simulink model "matrix5"  (R2018b)
settings: Solver=VariableStepAuto  StartTime=0.0  StopTime=1  RelTol=1e-6
model workspace (MAT data in the model file):
  A1 = 0.212
  A2 = 0.0033
  B1 = 0.311
  B2 = 0.0075
  C1 = 0.1
  C2 = 0.0084
  Ce1 = 0.27
  Ce2 = 0.12
  Cm1 = 0.36
  Cm2 = 0.12
  D1 = 0.1
  D2 = 0.001
  E1 = 0.1
  E2 = 0.001
  F1 = 0.1
  F2 = 0.001
  L1 = 0.00032
  L2 = 0.000194
  R1 = 0.32
  R2 = 0.485
  Xc2 = 0
  Yc2 = 0.0148
  g = 9.81
  m2 = 1.13085
settings Model: Creator=Sainquake  LastModifiedBy=Sainquake

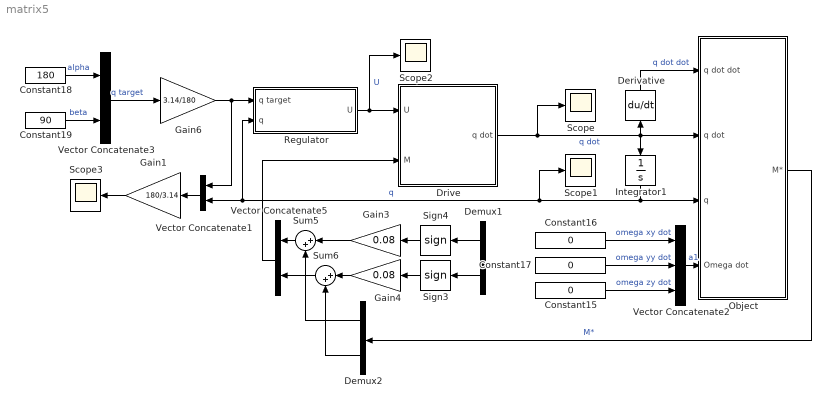
== system matrix5 ==
  Constant15 : Constant  Value=0
  Constant16 : Constant  Value=0
  Constant17 : Constant  Value=0
  Constant18 : Constant  Value=180
  Constant19 : Constant  Value=90
  Demux1 : Demux  Outputs=2
  Demux2 : Demux  Outputs=2
  Derivative : Derivative
  Drive : Subsystem
  Gain1 : Gain  Gain=180/3.14
  Gain3 : Gain  Gain=0.08
  Gain4 : Gain  Gain=0.08
  Gain6 : Gain  Gain=3.14/180
  Integrator1 : Integrator
  Object : Subsystem
  Regulator : Subsystem
  Scope{,1..3} (4 alike) : Scope
  Sign3 : Signum  ZeroCross=off
  Sign4 : Signum  ZeroCross=off
  Sum5 : Sum  Inputs=|++
  Sum6 : Sum  Inputs=|++
  Vector Concatenate1 : Concatenate
  Vector Concatenate2 : Concatenate  NumInputs=3
  Vector Concatenate3 : Concatenate
  Vector Concatenate5 : Concatenate
  wires:
  Integrator1/1 -> Regulator/2(q), Vector Concatenate1/2, Scope1/1, Object/3("q ")  "q"
  Constant15/1 -> Vector Concatenate2/3  "omega zy dot"
  Constant17/1 -> Vector Concatenate2/2  "omega yy dot"
  Constant16/1 -> Vector Concatenate2/1  "omega xy dot"
  Vector Concatenate2/1 -> Object/4(Omega dot)  "a1"
  Constant19/1 -> Vector Concatenate3/2  "beta"
  Constant18/1 -> Vector Concatenate3/1  "alpha"
  Drive/1(q dot) -> Integrator1/1, Object/2(q dot), Derivative/1, Scope/1  "q dot"
  Object/1(M*) -> Demux2/1  "M*"
  Regulator/1("U ") -> Scope2/1, Drive/1(U)  "U"
  Sign4/1 -> Gain3/1
  Sign3/1 -> Gain4/1
  Vector Concatenate5/1 -> Drive/2(M)
  Gain3/1 -> Sum5/1
  Demux2/1 -> Sum5/2
  Gain4/1 -> Sum6/1
  Demux2/2 -> Sum6/2
  Sum5/1 -> Vector Concatenate5/1
  Sum6/1 -> Vector Concatenate5/2
  Demux1/2 -> Sign3/1
  Demux1/1 -> Sign4/1
  Derivative/1 -> Object/1(q dot dot)  "q dot dot"
  Vector Concatenate3/1 -> Gain6/1  "q target"
  Vector Concatenate1/1 -> Gain1/1
  Gain1/1 -> Scope3/1
  Gain6/1 -> Vector Concatenate1/1, Regulator/1(q target)

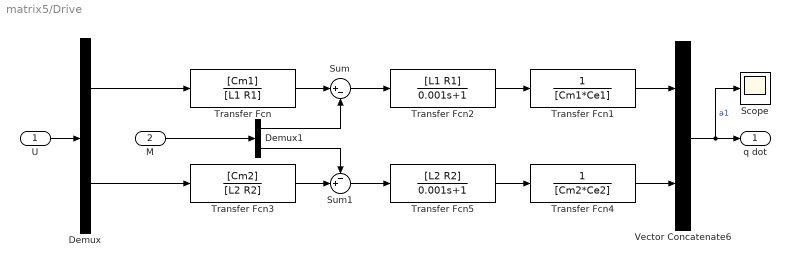
== system matrix5/Drive ==
  U : Inport
  M : Inport  Port=2
  Demux : Demux  Outputs=2
  Demux1 : Demux  Outputs=2
  Scope : Scope
  Sum : Sum  Inputs=|+-
  Sum1 : Sum  Inputs=-+|
  Transfer Fcn : TransferFcn  Numerator=[Cm1]  Denominator=[L1 R1]
  Transfer Fcn1 : TransferFcn  Numerator=1  Denominator=[Cm1*Ce1]
  Transfer Fcn2 : TransferFcn  Numerator=[L1 R1]  Denominator=[0.001 1]
  Transfer Fcn3 : TransferFcn  Numerator=[Cm2]  Denominator=[L2 R2]
  Transfer Fcn4 : TransferFcn  Numerator=1  Denominator=[Cm2*Ce2]
  Transfer Fcn5 : TransferFcn  Numerator=[L2 R2]  Denominator=[0.001 1]
  Vector Concatenate6 : Concatenate
  q dot : Outport
  wires:
  Sum/1 -> Transfer Fcn2/1
  Transfer Fcn3/1 -> Sum1/2
  Demux1/2 -> Sum1/1
  Demux/1 -> Transfer Fcn/1
  Vector Concatenate6/1 -> q dot/1, Scope/1  "a1"
  Transfer Fcn/1 -> Sum/1
  Transfer Fcn5/1 -> Transfer Fcn4/1
  Transfer Fcn2/1 -> Transfer Fcn1/1
  Demux1/1 -> Sum/2
  Demux/2 -> Transfer Fcn3/1
  Sum1/1 -> Transfer Fcn5/1
  Transfer Fcn1/1 -> Vector Concatenate6/1
  Transfer Fcn4/1 -> Vector Concatenate6/2
  U/1 -> Demux/1
  M/1 -> Demux1/1

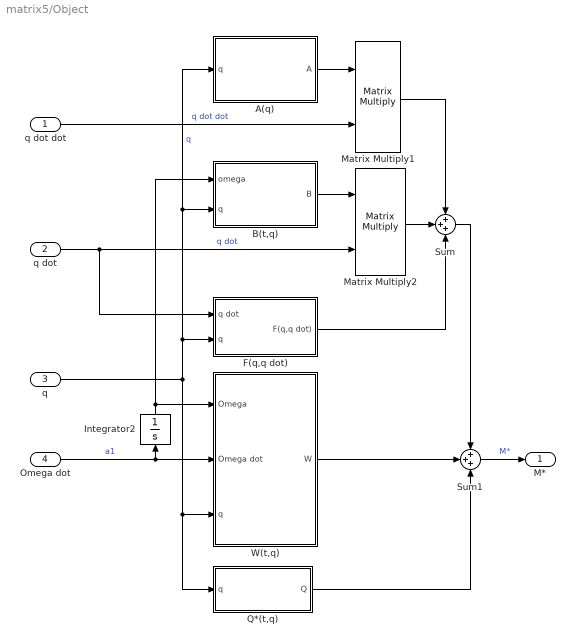
== system matrix5/Object ==
  q dot dot : Inport
  q dot : Inport  Port=2
  "q " : Inport  Port=3
  Omega dot : Inport  Port=4
  A(q) : Subsystem
  B(t,q) : Subsystem
  F(q,q dot) : Subsystem
  Integrator2 : Integrator
  Matrix Multiply1 : Product  Multiplication=Matrix(*)
  Matrix Multiply2 : Product  Multiplication=Matrix(*)
  Q*(t,q) : Subsystem
  Sum : Sum  Inputs=+++
  Sum1 : Sum  Inputs=+++
  W(t,q) : Subsystem
  M* : Outport
  wires:
  Integrator2/1 -> B(t,q)/1(omega), W(t,q)/1(Omega)
  Sum1/1 -> M*/1  "M*"
  A(q)/1(A) -> Matrix Multiply1/1
  q dot dot/1 -> Matrix Multiply1/2  "q dot dot"
  Omega dot/1 -> Integrator2/1, W(t,q)/2(Omega dot)  "a1"
  Sum/1 -> Sum1/1
  Matrix Multiply1/1 -> Sum/1
  Matrix Multiply2/1 -> Sum/2
  B(t,q)/1(B) -> Matrix Multiply2/1
  q dot/1 -> F(q,q dot)/1(q dot), Matrix Multiply2/2  "q dot"
  "q "/1 -> F(q,q dot)/2(q), B(t,q)/2(q), A(q)/1(q), Q*(t,q)/1(q), W(t,q)/3(q)  "q"
  W(t,q)/1(W) -> Sum1/2
  Q*(t,q)/1(Q) -> Sum1/3
  F(q,q dot)/1(F(q,q dot)) -> Sum/3

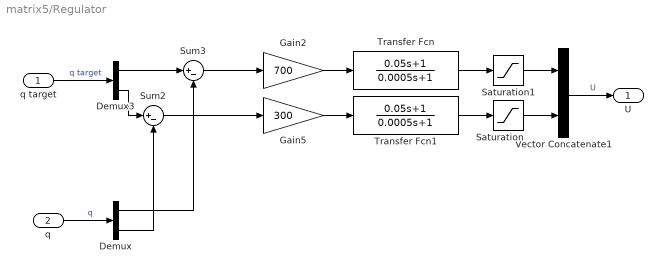
== system matrix5/Regulator ==
  q target : Inport
  q : Inport  Port=2
  Demux : Demux  Outputs=2
  Demux3 : Demux  Outputs=2
  Gain2 : Gain  Gain=700
  Gain5 : Gain  Gain=300
  Saturation : Saturate  UpperLimit=27  LowerLimit=-27  ZeroCross=off
  Saturation1 : Saturate  UpperLimit=27  LowerLimit=-27  ZeroCross=off
  Sum2 : Sum  Inputs=|+-
  Sum3 : Sum  Inputs=|+-
  Transfer Fcn : TransferFcn  Numerator=[0.05 1]  Denominator=[0.0005 1]
  Transfer Fcn1 : TransferFcn  Numerator=[0.05 1]  Denominator=[0.0005 1]
  Vector Concatenate1 : Concatenate
  "U " : Outport
  wires:
  Demux/1 -> Sum3/2
  Demux/2 -> Sum2/2
  Sum3/1 -> Gain2/1
  Transfer Fcn1/1 -> Saturation/1
  Saturation/1 -> Vector Concatenate1/2
  Sum2/1 -> Gain5/1
  Saturation1/1 -> Vector Concatenate1/1
  Demux3/2 -> Sum2/1
  Gain2/1 -> Transfer Fcn/1
  q target/1 -> Demux3/1  "q target"
  Gain5/1 -> Transfer Fcn1/1
  Demux3/1 -> Sum3/1
  Transfer Fcn/1 -> Saturation1/1
  q/1 -> Demux/1  "q"
  Vector Concatenate1/1 -> "U "/1  "U"

== system matrix5/Object/A(q) ==
  q : Inport
  B(beta) : Subsystem
  Constant10 : Constant  Value=C2
  Constant7 : Constant  Value=B1
  D(beta) : Subsystem
  Demux : Demux  Outputs=2
  Display5 : Display
  Gain : Gain  Gain=-1
  Sum : Sum  Inputs=|++
  Vector Concatenate1 : Concatenate
  Vector Concatenate2 : Concatenate
  Vector Concatenate6 : Concatenate  Mode=Multidimensional array  ConcatenateDimension=2
  A : Outport
  wires:
  q/1 -> Demux/1
  Constant7/1 -> Sum/2
  Vector Concatenate2/1 -> Vector Concatenate6/2  "a2"
  Sum/1 -> Vector Concatenate1/1  "a11"
  Constant10/1 -> Vector Concatenate2/2  "a22"
  Vector Concatenate1/1 -> Vector Concatenate6/1  "a1"
  B(beta)/1(B) -> Sum/1
  D(beta)/1(D) -> Gain/1
  Vector Concatenate6/1 -> A/1, Display5/1  "A"
  Gain/1 -> Vector Concatenate1/2, Vector Concatenate2/1  "a12"
  Demux/2 -> B(beta)/1(beta), D(beta)/1(beta)

== system matrix5/Object/B(t,q) ==
  omega : Inport
  q : Inport  Port=2
  Constant : Constant  Value=0
  Gain : Gain  Gain=-1
  Vector Concatenate3 : Concatenate
  Vector Concatenate4 : Concatenate
  Vector Concatenate5 : Concatenate  Mode=Multidimensional array  ConcatenateDimension=2
  b(t,alpha,beta) : Subsystem
  B : Outport
  wires:
  Vector Concatenate3/1 -> Vector Concatenate5/1  "a1"
  Vector Concatenate5/1 -> B/1  "A"
  Vector Concatenate4/1 -> Vector Concatenate5/2  "a2"
  b(t,alpha,beta)/1(b) -> Vector Concatenate3/2, Gain/1
  Gain/1 -> Vector Concatenate4/1
  Constant/1 -> Vector Concatenate4/2, Vector Concatenate3/1
  omega/1 -> b(t,alpha,beta)/1(omega)
  q/1 -> b(t,alpha,beta)/2(q)

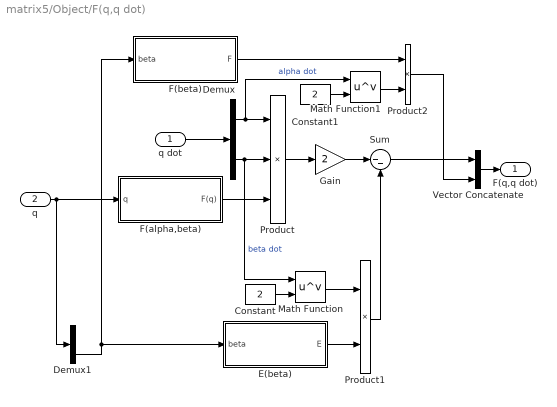
== system matrix5/Object/F(q,q dot) ==
  q dot : Inport
  q : Inport  Port=2
  Constant : Constant  Value=2
  Constant1 : Constant  Value=2
  Demux : Demux  Outputs=2
  Demux1 : Demux  Outputs=2
  E(beta) : Subsystem
  F(alpha,beta) : Subsystem
  F(beta) : Subsystem
  Gain : Gain  Gain=2
  Math Function : Math  Operator=pow  SaturateOnIntegerOverflow=on
  Math Function1 : Math  Operator=pow  SaturateOnIntegerOverflow=on
  Product : Product  Inputs=3
  Product1 : Product
  Product2 : Product
  Sum : Sum  Inputs=|--
  Vector Concatenate : Concatenate
  F(q,q dot) : Outport
  wires:
  q dot/1 -> Demux/1
  Product/1 -> Gain/1
  Demux/2 -> Product/2, Math Function/1  "beta dot"
  F(alpha,beta)/1(F(q)) -> Product/3
  q/1 -> Demux1/1, F(alpha,beta)/1(q)
  Constant/1 -> Math Function/2
  Math Function/1 -> Product1/1
  E(beta)/1(E) -> Product1/2
  Demux1/2 -> E(beta)/1(beta), F(beta)/1(beta)
  Gain/1 -> Sum/1
  Product1/1 -> Sum/2
  Constant1/1 -> Math Function1/2
  Demux/1 -> Product/1, Math Function1/1  "alpha dot"
  Math Function1/1 -> Product2/2
  F(beta)/1(F) -> Product2/1
  Product2/1 -> Vector Concatenate/2
  Sum/1 -> Vector Concatenate/1
  Vector Concatenate/1 -> F(q,q dot)/1

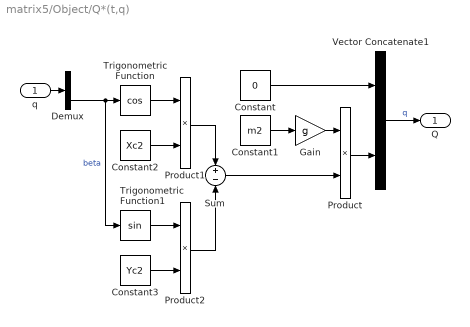
== system matrix5/Object/Q*(t,q) ==
  q : Inport
  Constant : Constant  Value=0
  Constant1 : Constant  Value=m2
  Constant2 : Constant  Value=Xc2
  Constant3 : Constant  Value=Yc2
  Demux : Demux  Outputs=2
  Gain : Gain  Gain=g
  Product : Product
  Product1 : Product
  Product2 : Product
  Sum : Sum  Inputs=+-
  Trigonometric Function : Trigonometry  Operator=cos
  Trigonometric Function1 : Trigonometry
  Vector Concatenate1 : Concatenate
  Q : Outport
  wires:
  Vector Concatenate1/1 -> Q/1  "q"
  Constant/1 -> Vector Concatenate1/1
  Product/1 -> Vector Concatenate1/2
  Gain/1 -> Product/1
  Constant1/1 -> Gain/1
  q/1 -> Demux/1
  Trigonometric Function/1 -> Product1/1
  Constant2/1 -> Product1/2
  Product1/1 -> Sum/1
  Constant3/1 -> Product2/2
  Demux/2 -> Trigonometric Function1/1, Trigonometric Function/1  "beta"
  Product2/1 -> Sum/2
  Trigonometric Function1/1 -> Product2/1
  Sum/1 -> Product/2

== system matrix5/Object/W(t,q) ==
  Omega : Inport
  Omega dot : Inport  Port=2
  q : Inport  Port=3
  Vector Concatenate : Concatenate
  "w alpha (t, q) " : Subsystem
  "w beta (t, q)" : Subsystem
  W : Outport
  wires:
  Omega/1 -> "w beta (t, q)"/1(Omega), "w alpha (t, q) "/1(Omega)
  Omega dot/1 -> "w beta (t, q)"/2(Omega dot), "w alpha (t, q) "/2(Omega dot)
  q/1 -> "w beta (t, q)"/3(q), "w alpha (t, q) "/3(q)
  "w alpha (t, q) "/1(w alpha) -> Vector Concatenate/1
  "w beta (t, q)"/1(w alpha) -> Vector Concatenate/2
  Vector Concatenate/1 -> W/1

== system matrix5/Object/A(q)/B(beta) ==
  beta : Inport
  Constant3 : Constant  Value=2
  Constant4 : Constant  Value=2
  Gain : Gain  Gain=B2
  Gain1 : Gain  Gain=A2
  Gain2 : Gain  Gain=F2
  Gain3 : Gain  Gain=2
  Math Function : Math  Operator=pow  SaturateOnIntegerOverflow=on
  Math Function1 : Math  Operator=pow  SaturateOnIntegerOverflow=on
  Sum : Sum  Inputs=++-
  Trigonometric Function : Trigonometry  Operator=cos
  Trigonometric Function1 : Trigonometry
  Trigonometric Function2 : Trigonometry
  B : Outport
  wires:
  beta/1 -> Gain3/1, Trigonometric Function1/1, Trigonometric Function/1
  Constant3/1 -> Math Function/2
  Trigonometric Function/1 -> Math Function/1
  Math Function/1 -> Gain/1
  Trigonometric Function1/1 -> Math Function1/1
  Math Function1/1 -> Gain1/1
  Constant4/1 -> Math Function1/2
  Trigonometric Function2/1 -> Gain2/1
  Gain3/1 -> Trigonometric Function2/1
  Gain1/1 -> Sum/2
  Gain/1 -> Sum/1
  Gain2/1 -> Sum/3
  Sum/1 -> B/1

== system matrix5/Object/A(q)/D(beta) ==
  beta : Inport
  Gain : Gain  Gain=D2
  Gain2 : Gain  Gain=E2
  Sum : Sum
  Trigonometric Function : Trigonometry  Operator=cos
  Trigonometric Function2 : Trigonometry
  D : Outport
  wires:
  Trigonometric Function/1 -> Gain/1
  Trigonometric Function2/1 -> Gain2/1
  beta/1 -> Trigonometric Function2/1, Trigonometric Function/1
  Gain/1 -> Sum/1
  Sum/1 -> D/1
  Gain2/1 -> Sum/2

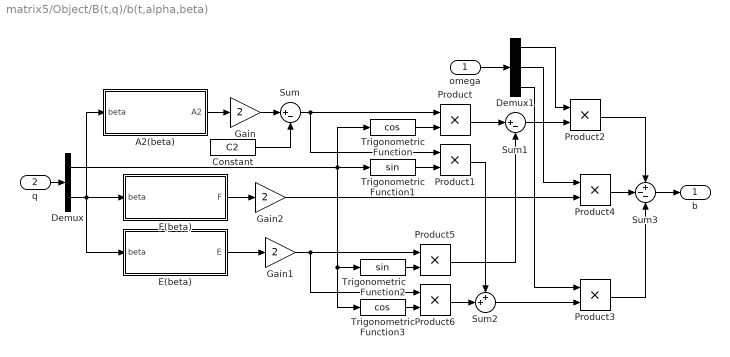
== system matrix5/Object/B(t,q)/b(t,alpha,beta) ==
  omega : Inport
  q : Inport  Port=2
  A2(beta) : Subsystem
  Constant : Constant  Value=C2
  Demux : Demux  Outputs=2
  Demux1 : Demux  Outputs=3
  E(beta) : Subsystem
  F(beta) : Subsystem
  Gain : Gain  Gain=2
  Gain1 : Gain  Gain=2
  Gain2 : Gain  Gain=2
  Product{,1..6} (7 alike) : Product
  Sum : Sum  Inputs=|+-
  Sum1 : Sum  Inputs=|+-
  Sum2 : Sum  Inputs=++|
  Sum3 : Sum  Inputs=+--
  Trigonometric Function : Trigonometry  Operator=cos
  Trigonometric Function1 : Trigonometry
  Trigonometric Function2 : Trigonometry
  Trigonometric Function3 : Trigonometry  Operator=cos
  b : Outport
  wires:
  q/1 -> Demux/1
  omega/1 -> Demux1/1
  A2(beta)/1(A2) -> Gain/1
  Constant/1 -> Sum/2
  Gain/1 -> Sum/1
  Sum/1 -> Product1/1, Product/1
  Trigonometric Function/1 -> Product/2
  Demux/1 -> Trigonometric Function3/1, Trigonometric Function2/1, Trigonometric Function1/1, Trigonometric Function/1
  Trigonometric Function1/1 -> Product1/2
  Demux1/1 -> Product2/1
  Trigonometric Function3/1 -> Product6/2
  Trigonometric Function2/1 -> Product5/2
  E(beta)/1(E) -> Gain1/1
  Gain1/1 -> Product6/1, Product5/1
  Demux/2 -> E(beta)/1(beta), A2(beta)/1(beta), F(beta)/1(beta)
  Product/1 -> Sum1/1
  Product5/1 -> Sum1/2
  Product6/1 -> Sum2/2
  Product1/1 -> Sum2/1
  Sum1/1 -> Product2/2
  F(beta)/1(F) -> Gain2/1
  Gain2/1 -> Product4/2
  Demux1/2 -> Product4/1
  Demux1/3 -> Product3/1
  Sum2/1 -> Product3/2
  Product2/1 -> Sum3/1
  Product4/1 -> Sum3/2
  Product3/1 -> Sum3/3
  Sum3/1 -> b/1

== system matrix5/Object/F(q,q dot)/E(beta) ==
  beta : Inport
  Gain : Gain  Gain=E2
  Gain2 : Gain  Gain=D2
  Sum : Sum  Inputs=+-
  Trigonometric Function : Trigonometry  Operator=cos
  Trigonometric Function2 : Trigonometry
  E : Outport
  wires:
  Trigonometric Function/1 -> Gain/1
  Trigonometric Function2/1 -> Gain2/1
  beta/1 -> Trigonometric Function2/1, Trigonometric Function/1
  Gain/1 -> Sum/1
  Sum/1 -> E/1
  Gain2/1 -> Sum/2

== system matrix5/Object/F(q,q dot)/F(alpha,beta) ==
  q : Inport
  Constant : Constant  Value=F1
  Constant1 : Constant  Value=D1
  D(beta) : Subsystem
  Demux : Demux  Outputs=2
  F(beta) : Subsystem
  Product : Product
  Product1 : Product
  Sum : Sum
  Sum1 : Sum  Inputs=|++
  Sum2 : Sum  Inputs=|++
  Trigonometric Function : Trigonometry  Operator=cos
  Trigonometric Function2 : Trigonometry
  F(q) : Outport
  wires:
  Trigonometric Function2/1 -> Product1/1
  Product1/1 -> Sum/2
  Trigonometric Function/1 -> Product/1
  Product/1 -> Sum/1
  Demux/1 -> Trigonometric Function2/1, Trigonometric Function/1
  Sum/1 -> F(q)/1
  F(beta)/1(F) -> Sum1/1
  Constant/1 -> Sum1/2
  Sum1/1 -> Product/2
  Demux/2 -> D(beta)/1(beta), F(beta)/1(beta)
  D(beta)/1(D) -> Sum2/1
  Constant1/1 -> Sum2/2
  Sum2/1 -> Product1/2
  q/1 -> Demux/1

== system matrix5/Object/F(q,q dot)/F(beta) ==
  beta : Inport
  Gain : Gain  Gain=F2
  Gain1 : Gain  Gain=2
  Gain2 : Gain  Gain=(A2-B2)/2
  Sum : Sum  Inputs=+-
  Trigonometric Function : Trigonometry  Operator=cos
  Trigonometric Function2 : Trigonometry
  F : Outport
  wires:
  Trigonometric Function/1 -> Gain/1
  Trigonometric Function2/1 -> Gain2/1
  beta/1 -> Trigonometric Function/1, Gain1/1
  Gain/1 -> Sum/1
  Sum/1 -> F/1
  Gain2/1 -> Sum/2
  Gain1/1 -> Trigonometric Function2/1

== system matrix5/Object/W(t,q)/w alpha (t, q)  ==
  Omega : Inport
  Omega dot : Inport  Port=2
  q : Inport  Port=3
  Sum : Sum  Inputs=|++
  bracket1 : Subsystem
  bracket2 : Subsystem
  w alpha : Outport
  wires:
  Omega dot/1 -> bracket1/1(Omega dot)
  q/1 -> bracket2/2(q), bracket1/2(q)
  Omega/1 -> bracket2/1(Omega)
  bracket1/1(Out1) -> Sum/1
  bracket2/1(Out1) -> Sum/2
  Sum/1 -> w alpha/1

== system matrix5/Object/W(t,q)/w beta (t, q) ==
  Omega : Inport
  Omega dot : Inport  Port=2
  q : Inport  Port=3
  Gain : Gain  Gain=1/2
  Sum : Sum  Inputs=|+-
  bracket1 : Subsystem
  bracket2 : Subsystem
  w alpha : Outport
  wires:
  Sum/1 -> w alpha/1
  bracket2/1(Out1) -> Gain/1
  bracket1/1(Out1) -> Sum/1
  Omega/1 -> bracket2/1(Omega)
  q/1 -> bracket1/2(q), bracket2/2(q)
  Omega dot/1 -> bracket1/1(Omega dot)
  Gain/1 -> Sum/2

== system matrix5/Object/B(t,q)/b(t,alpha,beta)/A2(beta) ==
  beta : Inport
  Gain : Gain  Gain=(A2-B2)/2
  Gain1 : Gain  Gain=2
  Gain2 : Gain  Gain=F2
  Sum : Sum
  Trigonometric Function : Trigonometry  Operator=cos
  Trigonometric Function2 : Trigonometry
  A2 : Outport
  wires:
  Trigonometric Function/1 -> Gain/1
  Trigonometric Function2/1 -> Gain2/1
  beta/1 -> Gain1/1
  Gain/1 -> Sum/1
  Sum/1 -> A2/1
  Gain2/1 -> Sum/2
  Gain1/1 -> Trigonometric Function2/1, Trigonometric Function/1

== system matrix5/Object/B(t,q)/b(t,alpha,beta)/E(beta) ==
  beta : Inport
  Gain : Gain  Gain=E2
  Gain2 : Gain  Gain=D2
  Sum : Sum  Inputs=+-
  Trigonometric Function : Trigonometry  Operator=cos
  Trigonometric Function2 : Trigonometry
  E : Outport
  wires:
  Trigonometric Function/1 -> Gain/1
  Trigonometric Function2/1 -> Gain2/1
  beta/1 -> Trigonometric Function2/1, Trigonometric Function/1
  Gain/1 -> Sum/1
  Sum/1 -> E/1
  Gain2/1 -> Sum/2

== system matrix5/Object/B(t,q)/b(t,alpha,beta)/F(beta) ==
  beta : Inport
  Gain : Gain  Gain=F2
  Gain1 : Gain  Gain=2
  Gain2 : Gain  Gain=(A2-B2)/2
  Sum : Sum  Inputs=+-
  Trigonometric Function : Trigonometry  Operator=cos
  Trigonometric Function2 : Trigonometry
  F : Outport
  wires:
  Trigonometric Function/1 -> Gain/1
  Trigonometric Function2/1 -> Gain2/1
  beta/1 -> Trigonometric Function/1, Gain1/1
  Gain/1 -> Sum/1
  Sum/1 -> F/1
  Gain2/1 -> Sum/2
  Gain1/1 -> Trigonometric Function2/1

== system matrix5/Object/F(q,q dot)/F(alpha,beta)/D(beta) ==
  beta : Inport
  Gain : Gain  Gain=D2
  Gain2 : Gain  Gain=E2
  Sum : Sum
  Trigonometric Function : Trigonometry  Operator=cos
  Trigonometric Function2 : Trigonometry
  D : Outport
  wires:
  Trigonometric Function/1 -> Gain/1
  Trigonometric Function2/1 -> Gain2/1
  beta/1 -> Trigonometric Function2/1, Trigonometric Function/1
  Gain/1 -> Sum/1
  Sum/1 -> D/1
  Gain2/1 -> Sum/2

== system matrix5/Object/F(q,q dot)/F(alpha,beta)/F(beta) ==
  beta : Inport
  Gain : Gain  Gain=F2
  Gain1 : Gain  Gain=2
  Gain2 : Gain  Gain=(A2-B2)/2
  Sum : Sum  Inputs=+-
  Trigonometric Function : Trigonometry  Operator=cos
  Trigonometric Function2 : Trigonometry
  F : Outport
  wires:
  Trigonometric Function/1 -> Gain/1
  Trigonometric Function2/1 -> Gain2/1
  beta/1 -> Trigonometric Function/1, Gain1/1
  Gain/1 -> Sum/1
  Sum/1 -> F/1
  Gain2/1 -> Sum/2
  Gain1/1 -> Trigonometric Function2/1

== system matrix5/Object/W(t,q)/w alpha (t, q) /bracket1 ==
  Omega dot : Inport
  q : Inport  Port=2
  B(beta) : Subsystem
  Constant7 : Constant  Value=B1
  D(alpha,beta) : Subsystem
  Demux : Demux  Outputs=3
  Demux1 : Demux  Outputs=2
  F(alpha,beta) : Subsystem
  Product : Product
  Product1 : Product
  Product2 : Product
  Sum : Sum  Inputs=|++
  Sum1 : Sum  Inputs=-+-
  Out1 : Outport
  wires:
  Demux/2 -> Product1/1
  F(alpha,beta)/1(F(q)) -> Product/2
  Demux/1 -> Product/1
  Product/1 -> Sum1/1
  D(alpha,beta)/1(D(q)) -> Product2/2
  Demux1/2 -> B(beta)/1(beta)
  Product2/1 -> Sum1/3
  Product1/1 -> Sum1/2
  B(beta)/1(B) -> Sum/1
  q/1 -> D(alpha,beta)/1(q), Demux1/1, F(alpha,beta)/1(q)
  Sum/1 -> Product1/2  "a11"
  Demux/3 -> Product2/1
  Constant7/1 -> Sum/2
  Omega dot/1 -> Demux/1
  Sum1/1 -> Out1/1

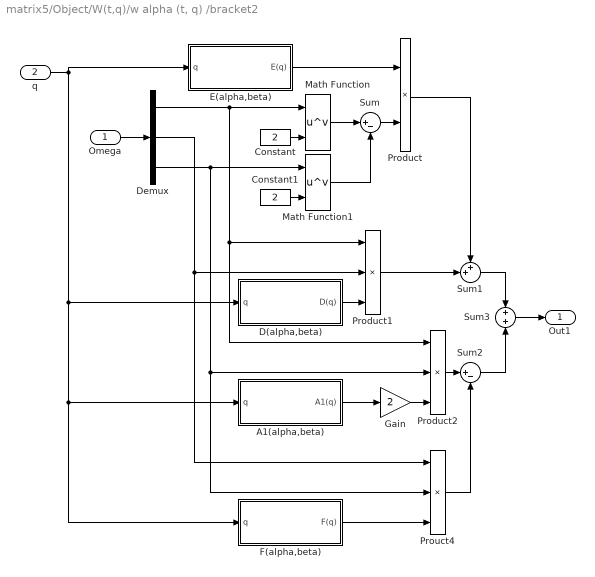
== system matrix5/Object/W(t,q)/w alpha (t, q) /bracket2 ==
  Omega : Inport
  q : Inport  Port=2
  A1(alpha,beta) : Subsystem
  Constant : Constant  Value=2
  Constant1 : Constant  Value=2
  D(alpha,beta) : Subsystem
  Demux : Demux  Outputs=3
  E(alpha,beta) : Subsystem
  F(alpha,beta) : Subsystem
  Gain : Gain  Gain=2
  Math Function : Math  Operator=pow  SaturateOnIntegerOverflow=on
  Math Function1 : Math  Operator=pow  SaturateOnIntegerOverflow=on
  Product : Product
  Product1 : Product  Inputs=3
  Product2 : Product  Inputs=3
  Prouct4 : Product  Inputs=3
  Sum : Sum  Inputs=|+-
  Sum1 : Sum  Inputs=++|
  Sum2 : Sum  Inputs=|+-
  Sum3 : Sum
  Out1 : Outport
  wires:
  Omega/1 -> Demux/1
  Constant/1 -> Math Function/2
  Demux/1 -> Product2/1, Product1/1, Math Function/1
  Constant1/1 -> Math Function1/2
  Math Function/1 -> Sum/1
  Math Function1/1 -> Sum/2
  E(alpha,beta)/1(E(q)) -> Product/1
  Sum/1 -> Product/2
  q/1 -> F(alpha,beta)/1(q), A1(alpha,beta)/1(q), D(alpha,beta)/1(q), E(alpha,beta)/1(q)
  Demux/2 -> Prouct4/1, Product1/2
  D(alpha,beta)/1(D(q)) -> Product1/3
  A1(alpha,beta)/1(A1(q)) -> Gain/1
  Gain/1 -> Product2/3
  F(alpha,beta)/1(F(q)) -> Prouct4/3
  Demux/3 -> Prouct4/2, Product2/2, Math Function1/1
  Product/1 -> Sum1/1
  Product1/1 -> Sum1/2
  Prouct4/1 -> Sum2/2
  Product2/1 -> Sum2/1
  Sum1/1 -> Sum3/1
  Sum2/1 -> Sum3/2
  Sum3/1 -> Out1/1

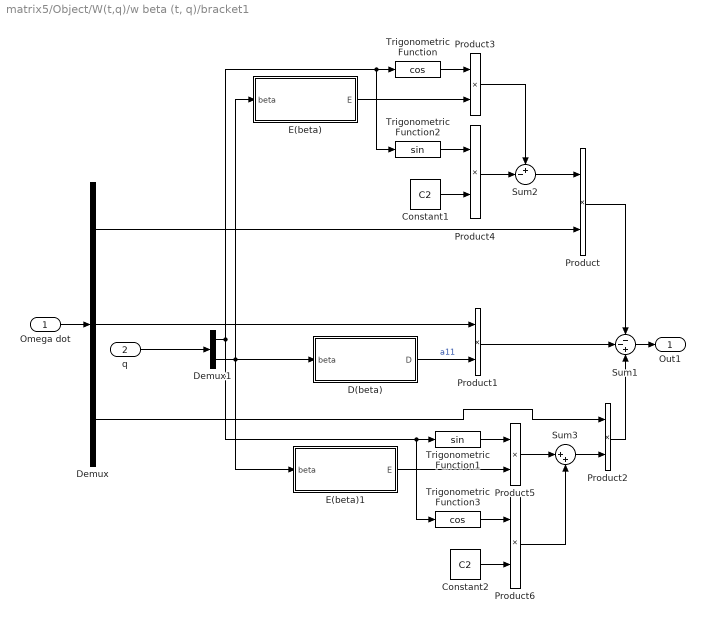
== system matrix5/Object/W(t,q)/w beta (t, q)/bracket1 ==
  Omega dot : Inport
  q : Inport  Port=2
  Constant1 : Constant  Value=C2
  Constant2 : Constant  Value=C2
  D(beta) : Subsystem
  Demux : Demux  Outputs=3
  Demux1 : Demux  Outputs=2
  E(beta) : Subsystem
  E(beta)1 : Subsystem
  Product{,1..6} (7 alike) : Product
  Sum1 : Sum  Inputs=--+
  Sum2 : Sum  Inputs=+-|
  Sum3 : Sum  Inputs=|++
  Trigonometric Function : Trigonometry  Operator=cos
  Trigonometric Function1 : Trigonometry
  Trigonometric Function2 : Trigonometry
  Trigonometric Function3 : Trigonometry  Operator=cos
  Out1 : Outport
  wires:
  Sum1/1 -> Out1/1
  Omega dot/1 -> Demux/1
  Demux/3 -> Product2/1
  D(beta)/1(D) -> Product1/2  "a11"
  q/1 -> Demux1/1
  Product1/1 -> Sum1/2
  Product2/1 -> Sum1/3
  Demux1/2 -> E(beta)1/1(beta), D(beta)/1(beta), E(beta)/1(beta)
  Product/1 -> Sum1/1
  Demux/1 -> Product/2
  Sum2/1 -> Product/1
  Demux/2 -> Product1/1
  Constant1/1 -> Product4/2
  Trigonometric Function/1 -> Product3/1
  Product4/1 -> Sum2/2
  Trigonometric Function2/1 -> Product4/1
  E(beta)/1(E) -> Product3/2
  Product3/1 -> Sum2/1
  Constant2/1 -> Product6/2
  Product5/1 -> Sum3/1
  Trigonometric Function3/1 -> Product6/1
  E(beta)1/1(E) -> Product5/2
  Sum3/1 -> Product2/2
  Trigonometric Function1/1 -> Product5/1
  Product6/1 -> Sum3/2
  Demux1/1 -> Trigonometric Function/1, Trigonometric Function2/1, Trigonometric Function1/1, Trigonometric Function3/1

== system matrix5/Object/W(t,q)/w beta (t, q)/bracket2 ==
  Omega : Inport
  q : Inport  Port=2
  Demux : Demux  Outputs=3
  Gain4 : Gain  Gain=2
  Product13 : Product
  Product14 : Product
  Product15 : Product
  Subsystem : Subsystem
  Subsystem1 : Subsystem
  Subsystem2 : Subsystem
  Subsystem3 : Subsystem
  Sum1 : Sum  Inputs=++|
  Sum8 : Sum  Inputs=+--
  Out1 : Outport
  wires:
  Demux/3 -> Product15/2, Product14/2
  Demux/2 -> Product15/1, Product13/2
  q/1 -> Subsystem/2(q), Subsystem3/1(q), Subsystem2/1(q), Subsystem1/1(q)
  Demux/1 -> Product14/1, Product13/1
  Omega/1 -> Subsystem/1(Omega), Demux/1
  Sum8/1 -> Gain4/1
  Gain4/1 -> Sum1/2
  Subsystem/1(Out1) -> Sum1/1
  Product13/1 -> Subsystem1/2(omega x omega y)
  Product14/1 -> Subsystem2/2(omega x omega z)
  Product15/1 -> Subsystem3/2(omega y omega z)
  Subsystem1/1(Out1) -> Sum8/1
  Subsystem2/1(Out1) -> Sum8/2
  Subsystem3/1(Out1) -> Sum8/3
  Sum1/1 -> Out1/1

== system matrix5/Object/W(t,q)/w alpha (t, q) /bracket1/B(beta) ==
  beta : Inport
  Constant3 : Constant  Value=2
  Constant4 : Constant  Value=2
  Gain : Gain  Gain=B2
  Gain1 : Gain  Gain=A2
  Gain2 : Gain  Gain=F2
  Gain3 : Gain  Gain=2
  Math Function : Math  Operator=pow  SaturateOnIntegerOverflow=on
  Math Function1 : Math  Operator=pow  SaturateOnIntegerOverflow=on
  Sum : Sum  Inputs=++-
  Trigonometric Function : Trigonometry  Operator=cos
  Trigonometric Function1 : Trigonometry
  Trigonometric Function2 : Trigonometry
  B : Outport
  wires:
  beta/1 -> Gain3/1, Trigonometric Function1/1, Trigonometric Function/1
  Constant3/1 -> Math Function/2
  Trigonometric Function/1 -> Math Function/1
  Math Function/1 -> Gain/1
  Trigonometric Function1/1 -> Math Function1/1
  Math Function1/1 -> Gain1/1
  Constant4/1 -> Math Function1/2
  Trigonometric Function2/1 -> Gain2/1
  Gain3/1 -> Trigonometric Function2/1
  Gain1/1 -> Sum/2
  Gain/1 -> Sum/1
  Gain2/1 -> Sum/3
  Sum/1 -> B/1

== system matrix5/Object/W(t,q)/w alpha (t, q) /bracket1/D(alpha,beta) ==
  q : Inport
  Constant : Constant  Value=F1
  Constant1 : Constant  Value=D1
  D(beta) : Subsystem
  Demux : Demux  Outputs=2
  F(beta) : Subsystem
  Product : Product
  Product1 : Product
  Sum : Sum  Inputs=-+
  Sum1 : Sum  Inputs=|++
  Sum2 : Sum  Inputs=|++
  Trigonometric Function : Trigonometry
  Trigonometric Function2 : Trigonometry  Operator=cos
  D(q) : Outport
  wires:
  Trigonometric Function2/1 -> Product1/1
  Product1/1 -> Sum/2
  Trigonometric Function/1 -> Product/1
  Product/1 -> Sum/1
  Demux/1 -> Trigonometric Function2/1, Trigonometric Function/1
  Sum/1 -> D(q)/1
  F(beta)/1(F) -> Sum1/1
  Constant/1 -> Sum1/2
  Sum1/1 -> Product/2
  Demux/2 -> D(beta)/1(beta), F(beta)/1(beta)
  D(beta)/1(D) -> Sum2/1
  Constant1/1 -> Sum2/2
  Sum2/1 -> Product1/2
  q/1 -> Demux/1

== system matrix5/Object/W(t,q)/w alpha (t, q) /bracket1/F(alpha,beta) ==
  q : Inport
  Constant : Constant  Value=F1
  Constant1 : Constant  Value=D1
  D(beta) : Subsystem
  Demux : Demux  Outputs=2
  F(beta) : Subsystem
  Product : Product
  Product1 : Product
  Sum : Sum
  Sum1 : Sum  Inputs=|++
  Sum2 : Sum  Inputs=|++
  Trigonometric Function : Trigonometry  Operator=cos
  Trigonometric Function2 : Trigonometry
  F(q) : Outport
  wires:
  Trigonometric Function2/1 -> Product1/1
  Product1/1 -> Sum/2
  Trigonometric Function/1 -> Product/1
  Product/1 -> Sum/1
  Demux/1 -> Trigonometric Function2/1, Trigonometric Function/1
  Sum/1 -> F(q)/1
  F(beta)/1(F) -> Sum1/1
  Constant/1 -> Sum1/2
  Sum1/1 -> Product/2
  Demux/2 -> D(beta)/1(beta), F(beta)/1(beta)
  D(beta)/1(D) -> Sum2/1
  Constant1/1 -> Sum2/2
  Sum2/1 -> Product1/2
  q/1 -> Demux/1

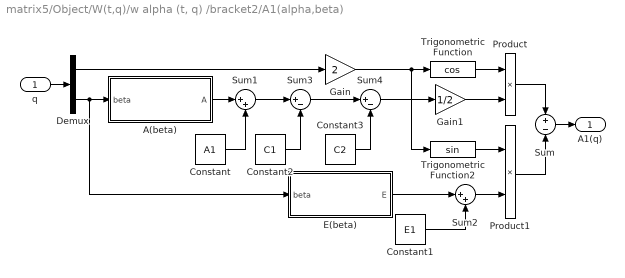
== system matrix5/Object/W(t,q)/w alpha (t, q) /bracket2/A1(alpha,beta) ==
  q : Inport
  A(beta) : Subsystem
  Constant : Constant  Value=A1
  Constant1 : Constant  Value=E1
  Constant2 : Constant  Value=C1
  Constant3 : Constant  Value=C2
  Demux : Demux  Outputs=2
  E(beta) : Subsystem
  Gain : Gain  Gain=2
  Gain1 : Gain  Gain=1/2
  Product : Product
  Product1 : Product
  Sum : Sum  Inputs=+-
  Sum1 : Sum  Inputs=|++
  Sum2 : Sum  Inputs=|++
  Sum3 : Sum  Inputs=|+-
  Sum4 : Sum  Inputs=|+-
  Trigonometric Function : Trigonometry  Operator=cos
  Trigonometric Function2 : Trigonometry
  A1(q) : Outport
  wires:
  Trigonometric Function2/1 -> Product1/1
  Product1/1 -> Sum/2
  Trigonometric Function/1 -> Product/1
  Product/1 -> Sum/1
  Demux/1 -> Gain/1
  Sum/1 -> A1(q)/1
  A(beta)/1(A) -> Sum1/1
  Constant/1 -> Sum1/2
  Sum1/1 -> Sum3/1
  Demux/2 -> E(beta)/1(beta), A(beta)/1(beta)
  E(beta)/1(E) -> Sum2/1
  Constant1/1 -> Sum2/2
  Sum2/1 -> Product1/2
  q/1 -> Demux/1
  Sum3/1 -> Sum4/1
  Sum4/1 -> Gain1/1
  Constant2/1 -> Sum3/2
  Constant3/1 -> Sum4/2
  Gain/1 -> Trigonometric Function2/1, Trigonometric Function/1
  Gain1/1 -> Product/2

== system matrix5/Object/W(t,q)/w alpha (t, q) /bracket2/D(alpha,beta) ==
  q : Inport
  Constant : Constant  Value=F1
  Constant1 : Constant  Value=D1
  D(beta) : Subsystem
  Demux : Demux  Outputs=2
  F(beta) : Subsystem
  Product : Product
  Product1 : Product
  Sum : Sum  Inputs=-+
  Sum1 : Sum  Inputs=|++
  Sum2 : Sum  Inputs=|++
  Trigonometric Function : Trigonometry
  Trigonometric Function2 : Trigonometry  Operator=cos
  D(q) : Outport
  wires:
  Trigonometric Function2/1 -> Product1/1
  Product1/1 -> Sum/2
  Trigonometric Function/1 -> Product/1
  Product/1 -> Sum/1
  Demux/1 -> Trigonometric Function2/1, Trigonometric Function/1
  Sum/1 -> D(q)/1
  F(beta)/1(F) -> Sum1/1
  Constant/1 -> Sum1/2
  Sum1/1 -> Product/2
  Demux/2 -> D(beta)/1(beta), F(beta)/1(beta)
  D(beta)/1(D) -> Sum2/1
  Constant1/1 -> Sum2/2
  Sum2/1 -> Product1/2
  q/1 -> Demux/1

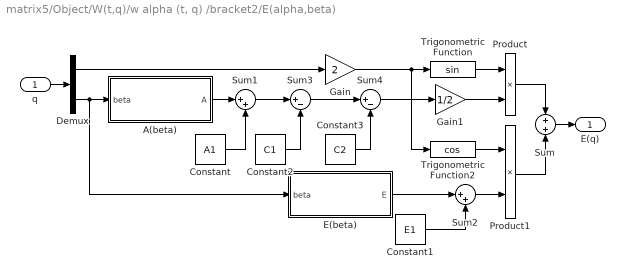
== system matrix5/Object/W(t,q)/w alpha (t, q) /bracket2/E(alpha,beta) ==
  q : Inport
  A(beta) : Subsystem
  Constant : Constant  Value=A1
  Constant1 : Constant  Value=E1
  Constant2 : Constant  Value=C1
  Constant3 : Constant  Value=C2
  Demux : Demux  Outputs=2
  E(beta) : Subsystem
  Gain : Gain  Gain=2
  Gain1 : Gain  Gain=1/2
  Product : Product
  Product1 : Product
  Sum : Sum
  Sum1 : Sum  Inputs=|++
  Sum2 : Sum  Inputs=|++
  Sum3 : Sum  Inputs=|+-
  Sum4 : Sum  Inputs=|+-
  Trigonometric Function : Trigonometry
  Trigonometric Function2 : Trigonometry  Operator=cos
  E(q) : Outport
  wires:
  Trigonometric Function2/1 -> Product1/1
  Product1/1 -> Sum/2
  Trigonometric Function/1 -> Product/1
  Product/1 -> Sum/1
  Demux/1 -> Gain/1
  Sum/1 -> E(q)/1
  A(beta)/1(A) -> Sum1/1
  Constant/1 -> Sum1/2
  Sum1/1 -> Sum3/1
  Demux/2 -> E(beta)/1(beta), A(beta)/1(beta)
  E(beta)/1(E) -> Sum2/1
  Constant1/1 -> Sum2/2
  Sum2/1 -> Product1/2
  q/1 -> Demux/1
  Sum3/1 -> Sum4/1
  Sum4/1 -> Gain1/1
  Constant2/1 -> Sum3/2
  Constant3/1 -> Sum4/2
  Gain/1 -> Trigonometric Function2/1, Trigonometric Function/1
  Gain1/1 -> Product/2

== system matrix5/Object/W(t,q)/w alpha (t, q) /bracket2/F(alpha,beta) ==
  q : Inport
  Constant : Constant  Value=F1
  Constant1 : Constant  Value=D1
  D(beta) : Subsystem
  Demux : Demux  Outputs=2
  F(beta) : Subsystem
  Product : Product
  Product1 : Product
  Sum : Sum
  Sum1 : Sum  Inputs=|++
  Sum2 : Sum  Inputs=|++
  Trigonometric Function : Trigonometry  Operator=cos
  Trigonometric Function2 : Trigonometry
  F(q) : Outport
  wires:
  Trigonometric Function2/1 -> Product1/1
  Product1/1 -> Sum/2
  Trigonometric Function/1 -> Product/1
  Product/1 -> Sum/1
  Demux/1 -> Trigonometric Function2/1, Trigonometric Function/1
  Sum/1 -> F(q)/1
  F(beta)/1(F) -> Sum1/1
  Constant/1 -> Sum1/2
  Sum1/1 -> Product/2
  Demux/2 -> D(beta)/1(beta), F(beta)/1(beta)
  D(beta)/1(D) -> Sum2/1
  Constant1/1 -> Sum2/2
  Sum2/1 -> Product1/2
  q/1 -> Demux/1

== system matrix5/Object/W(t,q)/w beta (t, q)/bracket1/D(beta) ==
  beta : Inport
  Gain : Gain  Gain=D2
  Gain2 : Gain  Gain=E2
  Sum : Sum
  Trigonometric Function : Trigonometry  Operator=cos
  Trigonometric Function2 : Trigonometry
  D : Outport
  wires:
  Gain2/1 -> Sum/2
  Sum/1 -> D/1
  Gain/1 -> Sum/1
  beta/1 -> Trigonometric Function/1, Trigonometric Function2/1
  Trigonometric Function2/1 -> Gain2/1
  Trigonometric Function/1 -> Gain/1

== system matrix5/Object/W(t,q)/w beta (t, q)/bracket1/E(beta) ==
  beta : Inport
  Gain : Gain  Gain=E2
  Gain2 : Gain  Gain=D2
  Sum : Sum  Inputs=+-
  Trigonometric Function : Trigonometry  Operator=cos
  Trigonometric Function2 : Trigonometry
  E : Outport
  wires:
  Gain2/1 -> Sum/2
  Sum/1 -> E/1
  Gain/1 -> Sum/1
  beta/1 -> Trigonometric Function/1, Trigonometric Function2/1
  Trigonometric Function2/1 -> Gain2/1
  Trigonometric Function/1 -> Gain/1

== system matrix5/Object/W(t,q)/w beta (t, q)/bracket1/E(beta)1 ==
  beta : Inport
  Gain : Gain  Gain=E2
  Gain2 : Gain  Gain=D2
  Sum : Sum  Inputs=+-
  Trigonometric Function : Trigonometry  Operator=cos
  Trigonometric Function2 : Trigonometry
  E : Outport
  wires:
  Gain2/1 -> Sum/2
  Sum/1 -> E/1
  Gain/1 -> Sum/1
  beta/1 -> Trigonometric Function/1, Trigonometric Function2/1
  Trigonometric Function2/1 -> Gain2/1
  Trigonometric Function/1 -> Gain/1

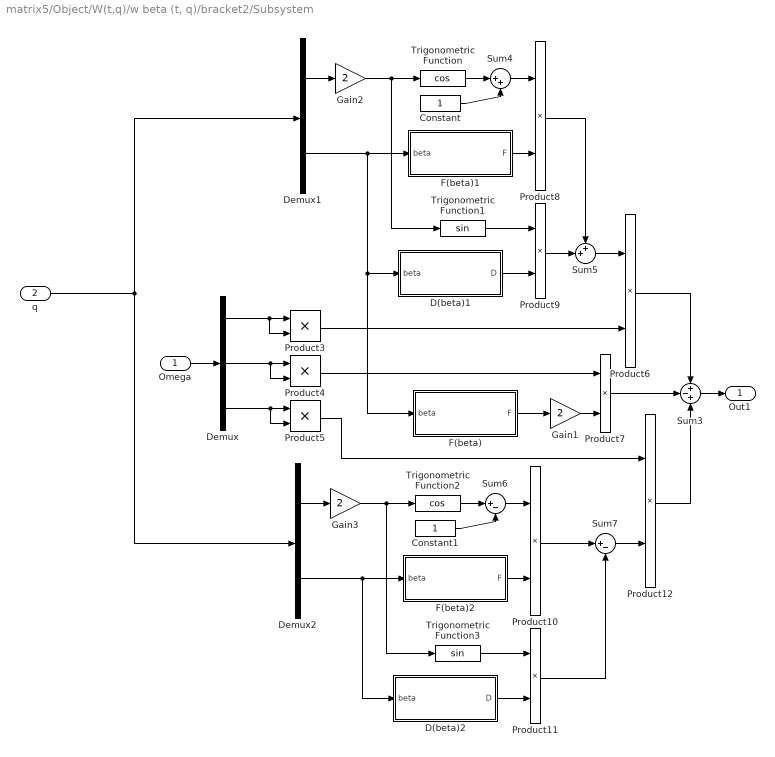
== system matrix5/Object/W(t,q)/w beta (t, q)/bracket2/Subsystem ==
  Omega : Inport
  q : Inport  Port=2
  Constant : Constant
  Constant1 : Constant
  D(beta)1 : Subsystem
  D(beta)2 : Subsystem
  Demux : Demux  Outputs=3
  Demux1 : Demux  Outputs=2
  Demux2 : Demux  Outputs=2
  F(beta) : Subsystem
  F(beta)1 : Subsystem
  F(beta)2 : Subsystem
  Gain1 : Gain  Gain=2
  Gain2 : Gain  Gain=2
  Gain3 : Gain  Gain=2
  Product{3..12} (10 alike) : Product
  Sum3 : Sum  Inputs=+-+
  Sum4 : Sum  Inputs=|++
  Sum5 : Sum  Inputs=++|
  Sum6 : Sum  Inputs=|+-
  Sum7 : Sum  Inputs=|+-
  Trigonometric Function : Trigonometry  Operator=cos
  Trigonometric Function1 : Trigonometry
  Trigonometric Function2 : Trigonometry  Operator=cos
  Trigonometric Function3 : Trigonometry
  Out1 : Outport
  wires:
  Trigonometric Function/1 -> Sum4/1
  Constant1/1 -> Sum6/2
  Demux2/2 -> D(beta)2/1(beta), F(beta)2/1(beta)
  Product10/1 -> Sum7/1
  Demux2/1 -> Gain3/1
  F(beta)2/1(F) -> Product10/2
  Gain3/1 -> Trigonometric Function3/1, Trigonometric Function2/1
  Sum6/1 -> Product10/1
  Trigonometric Function3/1 -> Product11/1
  D(beta)2/1(D) -> Product11/2
  Product12/1 -> Sum3/3
  Sum7/1 -> Product12/2
  Trigonometric Function2/1 -> Sum6/1
  Product8/1 -> Sum5/1
  Product9/1 -> Sum5/2
  Demux1/2 -> F(beta)/1(beta), D(beta)1/1(beta), F(beta)1/1(beta)
  Product6/1 -> Sum3/1
  F(beta)1/1(F) -> Product8/2
  D(beta)1/1(D) -> Product9/2
  Constant/1 -> Sum4/2
  Gain2/1 -> Trigonometric Function1/1, Trigonometric Function/1
  F(beta)/1(F) -> Gain1/1
  Product4/1 -> Product7/1
  Gain1/1 -> Product7/2
  Product3/1 -> Product6/2
  Product7/1 -> Sum3/2
  Product11/1 -> Sum7/2
  Demux1/1 -> Gain2/1
  Product5/1 -> Product12/1
  Trigonometric Function1/1 -> Product9/1
  Sum4/1 -> Product8/1
  Omega/1 -> Demux/1
  Demux/1 -> Product3/2, Product3/1
  Sum5/1 -> Product6/1
  Demux/2 -> Product4/2, Product4/1
  Demux/3 -> Product5/2, Product5/1
  q/1 -> Demux1/1, Demux2/1
  Sum3/1 -> Out1/1

== system matrix5/Object/W(t,q)/w beta (t, q)/bracket2/Subsystem1 ==
  q : Inport
  omega x omega y : Inport  Port=2
  A2(beta) : Subsystem
  Demux1 : Demux  Outputs=2
  E(beta) : Subsystem
  Gain1 : Gain  Gain=2
  Product : Product
  Product1 : Product
  Product3 : Product
  Sum : Sum  Inputs=+-
  Trigonometric Function : Trigonometry  Operator=cos
  Trigonometric Function1 : Trigonometry
  Out1 : Outport
  wires:
  Trigonometric Function/1 -> Product/1
  Demux1/2 -> E(beta)/1(beta), A2(beta)/1(beta)
  Product/1 -> Sum/1
  Gain1/1 -> Product/2
  Trigonometric Function1/1 -> Product3/2
  A2(beta)/1(A2) -> Gain1/1
  Demux1/1 -> Trigonometric Function1/1, Trigonometric Function/1
  E(beta)/1(E) -> Product3/1
  Product3/1 -> Sum/2
  Sum/1 -> Product1/1
  Product1/1 -> Out1/1
  q/1 -> Demux1/1
  omega x omega y/1 -> Product1/2

== system matrix5/Object/W(t,q)/w beta (t, q)/bracket2/Subsystem2 ==
  q : Inport
  omega x omega z : Inport  Port=2
  D(beta) : Subsystem
  Demux1 : Demux  Outputs=2
  F(beta) : Subsystem
  Gain : Gain  Gain=2
  Product : Product
  Product1 : Product
  Product3 : Product
  Sum : Sum  Inputs=+-
  Trigonometric Function : Trigonometry
  Trigonometric Function1 : Trigonometry  Operator=cos
  Out1 : Outport
  wires:
  omega x omega z/1 -> Product1/2
  q/1 -> Demux1/1
  Product1/1 -> Out1/1
  Sum/1 -> Product1/1
  Product3/1 -> Sum/2
  D(beta)/1(D) -> Product3/1
  Demux1/1 -> Gain/1
  Trigonometric Function1/1 -> Product3/2
  F(beta)/1(F) -> Product/2
  Product/1 -> Sum/1
  Trigonometric Function/1 -> Product/1
  Gain/1 -> Trigonometric Function/1, Trigonometric Function1/1
  Demux1/2 -> F(beta)/1(beta), D(beta)/1(beta)

== system matrix5/Object/W(t,q)/w beta (t, q)/bracket2/Subsystem3 ==
  q : Inport
  omega y omega z : Inport  Port=2
  A2(beta) : Subsystem
  Demux1 : Demux  Outputs=2
  E(beta) : Subsystem
  Gain1 : Gain  Gain=2
  Product : Product
  Product1 : Product
  Product3 : Product
  Sum : Sum
  Trigonometric Function : Trigonometry  Operator=cos
  Trigonometric Function1 : Trigonometry
  Out1 : Outport
  wires:
  omega y omega z/1 -> Product1/2
  q/1 -> Demux1/1
  Product1/1 -> Out1/1
  Sum/1 -> Product1/1
  Product3/1 -> Sum/2
  Gain1/1 -> Product3/1
  Demux1/1 -> Trigonometric Function/1, Trigonometric Function1/1
  Trigonometric Function1/1 -> Product3/2
  E(beta)/1(E) -> Product/2
  Product/1 -> Sum/1
  Demux1/2 -> A2(beta)/1(beta), E(beta)/1(beta)
  Trigonometric Function/1 -> Product/1
  A2(beta)/1(A2) -> Gain1/1

== system matrix5/Object/W(t,q)/w alpha (t, q) /bracket1/D(alpha,beta)/D(beta) ==
  beta : Inport
  Gain : Gain  Gain=D2
  Gain2 : Gain  Gain=E2
  Sum : Sum
  Trigonometric Function : Trigonometry  Operator=cos
  Trigonometric Function2 : Trigonometry
  D : Outport
  wires:
  Trigonometric Function/1 -> Gain/1
  Trigonometric Function2/1 -> Gain2/1
  beta/1 -> Trigonometric Function2/1, Trigonometric Function/1
  Gain/1 -> Sum/1
  Sum/1 -> D/1
  Gain2/1 -> Sum/2

== system matrix5/Object/W(t,q)/w alpha (t, q) /bracket1/D(alpha,beta)/F(beta) ==
  beta : Inport
  Gain : Gain  Gain=F2
  Gain1 : Gain  Gain=2
  Gain2 : Gain  Gain=(A2-B2)/2
  Sum : Sum  Inputs=+-
  Trigonometric Function : Trigonometry  Operator=cos
  Trigonometric Function2 : Trigonometry
  F : Outport
  wires:
  Trigonometric Function/1 -> Gain/1
  Trigonometric Function2/1 -> Gain2/1
  beta/1 -> Trigonometric Function/1, Gain1/1
  Gain/1 -> Sum/1
  Sum/1 -> F/1
  Gain2/1 -> Sum/2
  Gain1/1 -> Trigonometric Function2/1

== system matrix5/Object/W(t,q)/w alpha (t, q) /bracket1/F(alpha,beta)/D(beta) ==
  beta : Inport
  Gain : Gain  Gain=D2
  Gain2 : Gain  Gain=E2
  Sum : Sum
  Trigonometric Function : Trigonometry  Operator=cos
  Trigonometric Function2 : Trigonometry
  D : Outport
  wires:
  Trigonometric Function/1 -> Gain/1
  Trigonometric Function2/1 -> Gain2/1
  beta/1 -> Trigonometric Function2/1, Trigonometric Function/1
  Gain/1 -> Sum/1
  Sum/1 -> D/1
  Gain2/1 -> Sum/2

== system matrix5/Object/W(t,q)/w alpha (t, q) /bracket1/F(alpha,beta)/F(beta) ==
  beta : Inport
  Gain : Gain  Gain=F2
  Gain1 : Gain  Gain=2
  Gain2 : Gain  Gain=(A2-B2)/2
  Sum : Sum  Inputs=+-
  Trigonometric Function : Trigonometry  Operator=cos
  Trigonometric Function2 : Trigonometry
  F : Outport
  wires:
  Trigonometric Function/1 -> Gain/1
  Trigonometric Function2/1 -> Gain2/1
  beta/1 -> Trigonometric Function/1, Gain1/1
  Gain/1 -> Sum/1
  Sum/1 -> F/1
  Gain2/1 -> Sum/2
  Gain1/1 -> Trigonometric Function2/1

== system matrix5/Object/W(t,q)/w alpha (t, q) /bracket2/A1(alpha,beta)/A(beta) ==
  beta : Inport
  Constant : Constant  Value=2
  Constant1 : Constant  Value=2
  Gain : Gain  Gain=A2
  Gain1 : Gain  Gain=2
  Gain2 : Gain  Gain=F2
  Gain3 : Gain  Gain=B2
  Math Function : Math  Operator=pow  SaturateOnIntegerOverflow=on
  Math Function1 : Math  Operator=pow  SaturateOnIntegerOverflow=on
  Sum : Sum  Inputs=+++
  Trigonometric Function : Trigonometry  Operator=cos
  Trigonometric Function1 : Trigonometry
  Trigonometric Function2 : Trigonometry
  A : Outport
  wires:
  Trigonometric Function/1 -> Math Function/1
  Trigonometric Function2/1 -> Gain2/1
  Gain/1 -> Sum/1
  Sum/1 -> A/1
  Gain2/1 -> Sum/2
  Gain1/1 -> Trigonometric Function2/1
  Constant/1 -> Math Function/2
  Math Function/1 -> Gain/1
  Math Function1/1 -> Gain3/1
  Constant1/1 -> Math Function1/2
  beta/1 -> Trigonometric Function/1, Trigonometric Function1/1, Gain1/1
  Trigonometric Function1/1 -> Math Function1/1
  Gain3/1 -> Sum/3

== system matrix5/Object/W(t,q)/w alpha (t, q) /bracket2/A1(alpha,beta)/E(beta) ==
  beta : Inport
  Gain : Gain  Gain=E2
  Gain2 : Gain  Gain=D2
  Sum : Sum  Inputs=+-
  Trigonometric Function : Trigonometry  Operator=cos
  Trigonometric Function2 : Trigonometry
  E : Outport
  wires:
  Trigonometric Function/1 -> Gain/1
  Trigonometric Function2/1 -> Gain2/1
  beta/1 -> Trigonometric Function2/1, Trigonometric Function/1
  Gain/1 -> Sum/1
  Sum/1 -> E/1
  Gain2/1 -> Sum/2

== system matrix5/Object/W(t,q)/w alpha (t, q) /bracket2/D(alpha,beta)/D(beta) ==
  beta : Inport
  Gain : Gain  Gain=D2
  Gain2 : Gain  Gain=E2
  Sum : Sum
  Trigonometric Function : Trigonometry  Operator=cos
  Trigonometric Function2 : Trigonometry
  D : Outport
  wires:
  Trigonometric Function/1 -> Gain/1
  Trigonometric Function2/1 -> Gain2/1
  beta/1 -> Trigonometric Function2/1, Trigonometric Function/1
  Gain/1 -> Sum/1
  Sum/1 -> D/1
  Gain2/1 -> Sum/2

== system matrix5/Object/W(t,q)/w alpha (t, q) /bracket2/D(alpha,beta)/F(beta) ==
  beta : Inport
  Gain : Gain  Gain=F2
  Gain1 : Gain  Gain=2
  Gain2 : Gain  Gain=(A2-B2)/2
  Sum : Sum  Inputs=+-
  Trigonometric Function : Trigonometry  Operator=cos
  Trigonometric Function2 : Trigonometry
  F : Outport
  wires:
  Trigonometric Function/1 -> Gain/1
  Trigonometric Function2/1 -> Gain2/1
  beta/1 -> Trigonometric Function/1, Gain1/1
  Gain/1 -> Sum/1
  Sum/1 -> F/1
  Gain2/1 -> Sum/2
  Gain1/1 -> Trigonometric Function2/1

== system matrix5/Object/W(t,q)/w alpha (t, q) /bracket2/E(alpha,beta)/A(beta) ==
  beta : Inport
  Constant : Constant  Value=2
  Constant1 : Constant  Value=2
  Gain : Gain  Gain=A2
  Gain1 : Gain  Gain=2
  Gain2 : Gain  Gain=F2
  Gain3 : Gain  Gain=B2
  Math Function : Math  Operator=pow  SaturateOnIntegerOverflow=on
  Math Function1 : Math  Operator=pow  SaturateOnIntegerOverflow=on
  Sum : Sum  Inputs=+++
  Trigonometric Function : Trigonometry  Operator=cos
  Trigonometric Function1 : Trigonometry
  Trigonometric Function2 : Trigonometry
  A : Outport
  wires:
  Trigonometric Function/1 -> Math Function/1
  Trigonometric Function2/1 -> Gain2/1
  Gain/1 -> Sum/1
  Sum/1 -> A/1
  Gain2/1 -> Sum/2
  Gain1/1 -> Trigonometric Function2/1
  Constant/1 -> Math Function/2
  Math Function/1 -> Gain/1
  Math Function1/1 -> Gain3/1
  Constant1/1 -> Math Function1/2
  beta/1 -> Trigonometric Function/1, Trigonometric Function1/1, Gain1/1
  Trigonometric Function1/1 -> Math Function1/1
  Gain3/1 -> Sum/3

== system matrix5/Object/W(t,q)/w alpha (t, q) /bracket2/E(alpha,beta)/E(beta) ==
  beta : Inport
  Gain : Gain  Gain=E2
  Gain2 : Gain  Gain=D2
  Sum : Sum  Inputs=+-
  Trigonometric Function : Trigonometry  Operator=cos
  Trigonometric Function2 : Trigonometry
  E : Outport
  wires:
  Trigonometric Function/1 -> Gain/1
  Trigonometric Function2/1 -> Gain2/1
  beta/1 -> Trigonometric Function2/1, Trigonometric Function/1
  Gain/1 -> Sum/1
  Sum/1 -> E/1
  Gain2/1 -> Sum/2

== system matrix5/Object/W(t,q)/w alpha (t, q) /bracket2/F(alpha,beta)/D(beta) ==
  beta : Inport
  Gain : Gain  Gain=D2
  Gain2 : Gain  Gain=E2
  Sum : Sum
  Trigonometric Function : Trigonometry  Operator=cos
  Trigonometric Function2 : Trigonometry
  D : Outport
  wires:
  Trigonometric Function/1 -> Gain/1
  Trigonometric Function2/1 -> Gain2/1
  beta/1 -> Trigonometric Function2/1, Trigonometric Function/1
  Gain/1 -> Sum/1
  Sum/1 -> D/1
  Gain2/1 -> Sum/2

== system matrix5/Object/W(t,q)/w alpha (t, q) /bracket2/F(alpha,beta)/F(beta) ==
  beta : Inport
  Gain : Gain  Gain=F2
  Gain1 : Gain  Gain=2
  Gain2 : Gain  Gain=(A2-B2)/2
  Sum : Sum  Inputs=+-
  Trigonometric Function : Trigonometry  Operator=cos
  Trigonometric Function2 : Trigonometry
  F : Outport
  wires:
  Trigonometric Function/1 -> Gain/1
  Trigonometric Function2/1 -> Gain2/1
  beta/1 -> Trigonometric Function/1, Gain1/1
  Gain/1 -> Sum/1
  Sum/1 -> F/1
  Gain2/1 -> Sum/2
  Gain1/1 -> Trigonometric Function2/1

== system matrix5/Object/W(t,q)/w beta (t, q)/bracket2/Subsystem/D(beta)1 ==
  beta : Inport
  Gain : Gain  Gain=D2
  Gain2 : Gain  Gain=E2
  Sum : Sum
  Trigonometric Function : Trigonometry  Operator=cos
  Trigonometric Function2 : Trigonometry
  D : Outport
  wires:
  Trigonometric Function/1 -> Gain/1
  Trigonometric Function2/1 -> Gain2/1
  beta/1 -> Trigonometric Function2/1, Trigonometric Function/1
  Gain/1 -> Sum/1
  Sum/1 -> D/1
  Gain2/1 -> Sum/2

== system matrix5/Object/W(t,q)/w beta (t, q)/bracket2/Subsystem/D(beta)2 ==
  beta : Inport
  Gain : Gain  Gain=D2
  Gain2 : Gain  Gain=E2
  Sum : Sum
  Trigonometric Function : Trigonometry  Operator=cos
  Trigonometric Function2 : Trigonometry
  D : Outport
  wires:
  Trigonometric Function/1 -> Gain/1
  Trigonometric Function2/1 -> Gain2/1
  beta/1 -> Trigonometric Function2/1, Trigonometric Function/1
  Gain/1 -> Sum/1
  Sum/1 -> D/1
  Gain2/1 -> Sum/2

== system matrix5/Object/W(t,q)/w beta (t, q)/bracket2/Subsystem/F(beta) ==
  beta : Inport
  Gain : Gain  Gain=F2
  Gain1 : Gain  Gain=2
  Gain2 : Gain  Gain=(A2-B2)/2
  Sum : Sum  Inputs=+-
  Trigonometric Function : Trigonometry  Operator=cos
  Trigonometric Function2 : Trigonometry
  F : Outport
  wires:
  Gain1/1 -> Trigonometric Function2/1
  Gain2/1 -> Sum/2
  Sum/1 -> F/1
  Gain/1 -> Sum/1
  beta/1 -> Gain1/1, Trigonometric Function/1
  Trigonometric Function2/1 -> Gain2/1
  Trigonometric Function/1 -> Gain/1

== system matrix5/Object/W(t,q)/w beta (t, q)/bracket2/Subsystem/F(beta)1 ==
  beta : Inport
  Gain : Gain  Gain=F2
  Gain1 : Gain  Gain=2
  Gain2 : Gain  Gain=(A2-B2)/2
  Sum : Sum  Inputs=+-
  Trigonometric Function : Trigonometry  Operator=cos
  Trigonometric Function2 : Trigonometry
  F : Outport
  wires:
  Trigonometric Function/1 -> Gain/1
  Trigonometric Function2/1 -> Gain2/1
  beta/1 -> Trigonometric Function/1, Gain1/1
  Gain/1 -> Sum/1
  Sum/1 -> F/1
  Gain2/1 -> Sum/2
  Gain1/1 -> Trigonometric Function2/1

== system matrix5/Object/W(t,q)/w beta (t, q)/bracket2/Subsystem/F(beta)2 ==
  beta : Inport
  Gain : Gain  Gain=F2
  Gain1 : Gain  Gain=2
  Gain2 : Gain  Gain=(A2-B2)/2
  Sum : Sum  Inputs=+-
  Trigonometric Function : Trigonometry  Operator=cos
  Trigonometric Function2 : Trigonometry
  F : Outport
  wires:
  Trigonometric Function/1 -> Gain/1
  Trigonometric Function2/1 -> Gain2/1
  beta/1 -> Trigonometric Function/1, Gain1/1
  Gain/1 -> Sum/1
  Sum/1 -> F/1
  Gain2/1 -> Sum/2
  Gain1/1 -> Trigonometric Function2/1

== system matrix5/Object/W(t,q)/w beta (t, q)/bracket2/Subsystem1/A2(beta) ==
  beta : Inport
  Gain : Gain  Gain=A2-B2
  Gain1 : Gain  Gain=2
  Gain2 : Gain  Gain=F2
  Gain3 : Gain  Gain=1/2
  Sum : Sum
  Trigonometric Function : Trigonometry  Operator=cos
  Trigonometric Function2 : Trigonometry
  A2 : Outport
  wires:
  Trigonometric Function/1 -> Gain/1
  Trigonometric Function2/1 -> Gain2/1
  beta/1 -> Gain1/1
  Gain/1 -> Gain3/1
  Sum/1 -> A2/1
  Gain2/1 -> Sum/2
  Gain1/1 -> Trigonometric Function/1, Trigonometric Function2/1
  Gain3/1 -> Sum/1

== system matrix5/Object/W(t,q)/w beta (t, q)/bracket2/Subsystem1/E(beta) ==
  beta : Inport
  Gain : Gain  Gain=E2
  Gain2 : Gain  Gain=D2
  Sum : Sum  Inputs=+-
  Trigonometric Function : Trigonometry  Operator=cos
  Trigonometric Function2 : Trigonometry
  E : Outport
  wires:
  Gain2/1 -> Sum/2
  Sum/1 -> E/1
  Gain/1 -> Sum/1
  beta/1 -> Trigonometric Function/1, Trigonometric Function2/1
  Trigonometric Function2/1 -> Gain2/1
  Trigonometric Function/1 -> Gain/1

== system matrix5/Object/W(t,q)/w beta (t, q)/bracket2/Subsystem2/D(beta) ==
  beta : Inport
  Gain : Gain  Gain=D2
  Gain2 : Gain  Gain=E2
  Sum : Sum
  Trigonometric Function : Trigonometry  Operator=cos
  Trigonometric Function2 : Trigonometry
  D : Outport
  wires:
  Gain2/1 -> Sum/2
  Sum/1 -> D/1
  Gain/1 -> Sum/1
  beta/1 -> Trigonometric Function/1, Trigonometric Function2/1
  Trigonometric Function2/1 -> Gain2/1
  Trigonometric Function/1 -> Gain/1

== system matrix5/Object/W(t,q)/w beta (t, q)/bracket2/Subsystem2/F(beta) ==
  beta : Inport
  Gain : Gain  Gain=F2
  Gain1 : Gain  Gain=2
  Gain2 : Gain  Gain=(A2-B2)/2
  Sum : Sum  Inputs=+-
  Trigonometric Function : Trigonometry  Operator=cos
  Trigonometric Function2 : Trigonometry
  F : Outport
  wires:
  Trigonometric Function/1 -> Gain/1
  Trigonometric Function2/1 -> Gain2/1
  beta/1 -> Trigonometric Function/1, Gain1/1
  Gain/1 -> Sum/1
  Sum/1 -> F/1
  Gain2/1 -> Sum/2
  Gain1/1 -> Trigonometric Function2/1

== system matrix5/Object/W(t,q)/w beta (t, q)/bracket2/Subsystem3/A2(beta) ==
  beta : Inport
  Gain : Gain  Gain=A2-B2
  Gain1 : Gain  Gain=2
  Gain2 : Gain  Gain=F2
  Gain3 : Gain  Gain=1/2
  Sum : Sum
  Trigonometric Function : Trigonometry  Operator=cos
  Trigonometric Function2 : Trigonometry
  A2 : Outport
  wires:
  Gain3/1 -> Sum/1
  Gain1/1 -> Trigonometric Function2/1, Trigonometric Function/1
  Gain2/1 -> Sum/2
  Sum/1 -> A2/1
  Gain/1 -> Gain3/1
  beta/1 -> Gain1/1
  Trigonometric Function2/1 -> Gain2/1
  Trigonometric Function/1 -> Gain/1

== system matrix5/Object/W(t,q)/w beta (t, q)/bracket2/Subsystem3/E(beta) ==
  beta : Inport
  Gain : Gain  Gain=E2
  Gain2 : Gain  Gain=D2
  Sum : Sum  Inputs=+-
  Trigonometric Function : Trigonometry  Operator=cos
  Trigonometric Function2 : Trigonometry
  E : Outport
  wires:
  Trigonometric Function/1 -> Gain/1
  Trigonometric Function2/1 -> Gain2/1
  beta/1 -> Trigonometric Function2/1, Trigonometric Function/1
  Gain/1 -> Sum/1
  Sum/1 -> E/1
  Gain2/1 -> Sum/2
